simulink model "NestedBus"  (R2020a)
settings: configuration reference "CigreConfig" (kept outside this file)
undefined symbols (not defined in the file or in its folder): DiscIntNeverNeededParam
settings Model: DataDictionary=Definitions.sldd  Creator=toma  LastModifiedBy=toma
settings ConfigSetRef: SourceName=CigreConfig

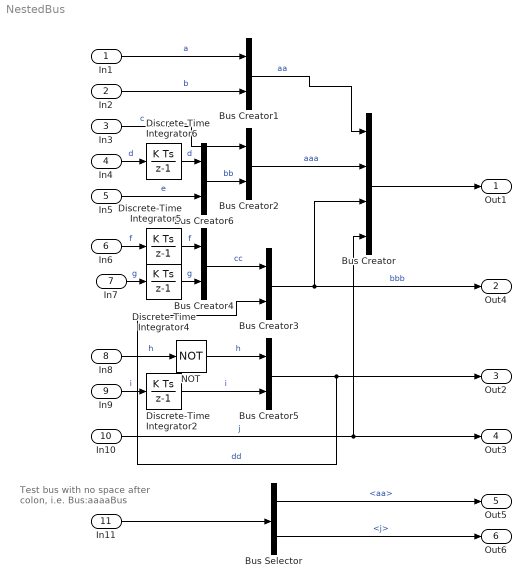
== system NestedBus ==
  note: Test bus with no space
      | after colon, i.e. Bus:aaaaBus
  In1 : Inport  OutDataTypeStr=Enum: MyEnum
  In2 : Inport  Port=2
  In3 : Inport  Port=3
  In4 : Inport  Port=4
  In5 : Inport  Port=5
  In6 : Inport  Port=6
  In7 : Inport  Port=7
  In8 : Inport  Port=8
  In9 : Inport  Port=9
  In10 : Inport  Port=10  OutDataTypeStr=Enum: MyEnum
  In11 : Inport  Port=11  OutDataTypeStr=Bus:aaaaBus  Interpolate=off  BusOutputAsStruct=on
  Bus Creator : BusCreator  Inputs=4  OutDataTypeStr=Bus: aaaaBus
  Bus Creator1 : BusCreator  Inputs=2  OutDataTypeStr=Bus: aaBus
  Bus Creator2 : BusCreator  Inputs=2  OutDataTypeStr=Bus: aaaBus
  Bus Creator3 : BusCreator  Inputs=2  OutDataTypeStr=Bus: bbbBus
  Bus Creator4 : BusCreator  Inputs=2  OutDataTypeStr=Bus: ccBus
  Bus Creator5 : BusCreator  Inputs=2  OutDataTypeStr=Bus: ddBus
  Bus Creator6 : BusCreator  Inputs=2  OutDataTypeStr=Bus: bbBus
  Bus Selector : BusSelector  OutputSignals=aa,j
  Discrete-Time Integrator2 : DiscreteIntegrator  InitialCondition=4  SampleTime=-1  ICPrevOutput=DiscIntNeverNeededParam  ICPrevScaledInput=DiscIntNeverNeededParam
  Discrete-Time Integrator4 : DiscreteIntegrator  InitialCondition=2  SampleTime=-1  ICPrevOutput=DiscIntNeverNeededParam  ICPrevScaledInput=DiscIntNeverNeededParam
  Discrete-Time Integrator5 : DiscreteIntegrator  InitialCondition=[1 2; 3 4]  SampleTime=-1  ICPrevOutput=DiscIntNeverNeededParam  ICPrevScaledInput=DiscIntNeverNeededParam
  Discrete-Time Integrator6 : DiscreteIntegrator  InitialCondition=1  SampleTime=-1  ICPrevOutput=DiscIntNeverNeededParam  ICPrevScaledInput=DiscIntNeverNeededParam
  NOT : Logic  Operator=NOT  IconShape=distinctive  AllPortsSameDT=off  OutDataTypeStr=boolean
  Out1 : Outport  OutDataTypeStr=Bus: aaaaBus
  Out4 : Outport  Port=2  OutDataTypeStr=Bus: bbbBus
  Out2 : Outport  Port=3  OutDataTypeStr=Bus: ddBus
  Out3 : Outport  Port=4  OutDataTypeStr=Enum: MyEnum
  Out5 : Outport  Port=5  OutDataTypeStr=Bus: aaBus
  Out6 : Outport  Port=6  OutDataTypeStr=Enum: MyEnum
  wires:
  Bus Creator2/1 -> Bus Creator/2  "aaa"
  In11/1 -> Bus Selector/1
  In8/1 -> NOT/1  "h"
  Bus Creator1/1 -> Bus Creator/1  "aa"
  In7/1 -> Discrete-Time Integrator4/1  "g"
  In4/1 -> Discrete-Time Integrator6/1  "d"
  Bus Creator3/1 -> Out4/1, Bus Creator/3  "bbb"
  In5/1 -> Bus Creator6/2  "e"
  In6/1 -> Discrete-Time Integrator5/1  "f"
  In9/1 -> Discrete-Time Integrator2/1  "i"
  In1/1 -> Bus Creator1/1  "a"
  In2/1 -> Bus Creator1/2  "b"
  In3/1 -> Bus Creator2/1  "c"
  Bus Creator6/1 -> Bus Creator2/2  "bb"
  Bus Creator4/1 -> Bus Creator3/1  "cc"
  Bus Creator5/1 -> Out2/1, Bus Creator3/2  "dd"
  Bus Selector/1 -> Out5/1  "<aa>"
  Bus Selector/2 -> Out6/1  "<j>"
  In10/1 -> Out3/1, Bus Creator/4  "j"
  Bus Creator/1 -> Out1/1
  Discrete-Time Integrator2/1 -> Bus Creator5/2  "i"
  NOT/1 -> Bus Creator5/1  "h"
  Discrete-Time Integrator4/1 -> Bus Creator4/2  "g"
  Discrete-Time Integrator5/1 -> Bus Creator4/1  "f"
  Discrete-Time Integrator6/1 -> Bus Creator6/1  "d"
